simulink model "vehicle_psd"  (R2017a)
settings: Solver=FixedStepDiscrete  StartTime=0.0  StopTime=5e3  FixedStep=abs(Ts)  RelTol=1e-3
InitFcn:
  | if ~exist('Ts')
  |     Ts = 1;
  | end
undefined symbols (not defined in the file or in its folder): elvio_cycle_eu_nedc
libraries: elvio x19
settings Model: Creator=tstef  LastModifiedBy=thomas
settings OptimizationCC: LifeSpan=inf
settings DebuggingCC: SFExecutionAtInitializationDiag=none

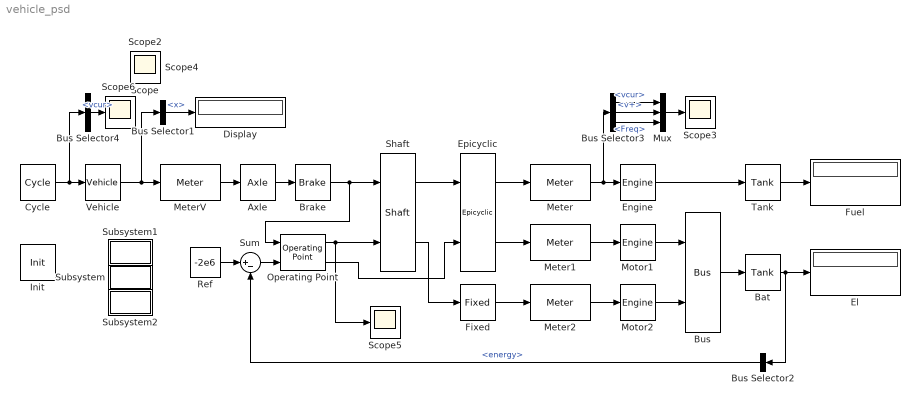
== system vehicle_psd ==
  Axle : elvio/Drive/Axle  radius=0.3  ratio=4  factor=0.1  FromTag1=Axle1  GotoTag1=MeterV1
  Bat : elvio/Drive/Tank  GotoTag1=Bus1
  Brake : elvio/Drive/Brake  Tbrake=5000  FromTag1=Brake1  GotoTag1=Axle1
  Bus : elvio/Drive/Bus  GotoTag1=Motor11  GotoTag2=Motor21  FromTag1=Bus1
  Bus Selector1 : BusSelector  OutputSignals=info.x
  Bus Selector2 : BusSelector  OutputSignals=energy
  Bus Selector3 : BusSelector  OutputSignals=vcur,v+,Freq
  Bus Selector4 : BusSelector  OutputSignals=vcur
  Cycle : elvio/Drive/Cycle  data=elvio_cycle_eu_nedc()
  Display : Display
  El : Display
  Engine : elvio/Drive/Engine  Tmax=110  Tmin=-12  Tfrict=12  Ploss=1000  lossf=1.1  lossnorm=500e3  lossR=0.2  FromTag1=Engine1  GotoTag1=Meter1
  Epicyclic : elvio/Drive/Epicyclic  a=0.4  FromTag1=Epicyclic1  FromTag2=Epicyclic2  GotoTag1=Shaft1
  Fixed : elvio/Drive/Fixed  gear=2  factor=0.1  FromTag1=Fixed1  GotoTag1=Shaft2
  Fuel : Display
  Init : elvio/Drive/Init  Ts0=1
  Meter : elvio/Drive/Meter  FromTag1=Meter1  GotoTag1=Epicyclic1
  Meter1 : elvio/Drive/Meter  FromTag1=Meter11  GotoTag1=Epicyclic2
  Meter2 : elvio/Drive/Meter  FromTag1=Meter21  GotoTag1=Fixed1
  MeterV : elvio/Drive/Meter  FromTag1=MeterV1  GotoTag1=Vehicle1
  Motor1 : elvio/Drive/Engine  Tmax=60  Tmin=-60  Tfrict=0.2  Ploss=100  lossf=0.01  lossnorm=2e6  lossR=0.05  FromTag1=Motor11  GotoTag1=Meter11
  Motor2 : elvio/Drive/Engine  Tmax=60  Tmin=-60  Tfrict=0.2  Ploss=100  lossf=0.01  lossnorm=2e6  lossR=0.05  FromTag1=Motor21  GotoTag1=Meter21
  Mux : Mux  Inputs=3
  Operating Point : elvio/Drive/Operating Point  a=0.4  T=1000  Pk=0.5  Pbias=5e3  Pmin=4e3  vmin=100  vmax=400  Tmin=10  Tmax=80
  Ref : Constant  Value=-2e6
  Scope{,2..6} (6 alike) : Scope
      Scope4 mask Display: disp('1.484e+07')
  Shaft : elvio/Drive/Shaft  FromTag1=Shaft1  FromTag2=Shaft2  GotoTag1=Brake1
  Subsystem : Subsystem
      settings: OpenFcn=elvio_plot_scatter(logsout);
      mask Display: disp('Scatter')
  Subsystem1 : Subsystem
      settings: OpenFcn=elvio_plot_energy(logsout);
      mask Display: disp('Energy')
  Subsystem2 : Subsystem
      settings: OpenFcn=elvio_plot_sources(logsout);
      mask Display: disp('Sources')
  Sum : Sum  Inputs=|+-
  Tank : elvio/Drive/Tank  GotoTag1=Engine1
  Vehicle : elvio/Drive/Vehicle  m=1200  Froll=150  Aeff=0.3:0.025:0.4  n=[1 5]  FromTag1=Vehicle1
  wires:
  Vehicle/1 -> MeterV/1, Bus Selector1/1
  Engine/1 -> Tank/1
  Tank/1 -> Fuel/1
  Operating Point/1 -> Scope5/1, Shaft/2
  Bus/1 -> Bat/1
  Motor1/1 -> Bus/1
  Motor2/1 -> Bus/2
  Shaft/1 -> Epicyclic/1
  Epicyclic/1 -> Meter/1
  Operating Point/2 -> Epicyclic/2
  Bat/1 -> Bus Selector2/1, El/1
  Bus Selector1/1 -> Display/1  "<x>"
  Shaft/2 -> Fixed/1
  Fixed/1 -> Meter2/1
  Epicyclic/2 -> Meter1/1
  Meter1/1 -> Motor1/1
  Meter2/1 -> Motor2/1
  MeterV/1 -> Axle/1
  Bus Selector3/3 -> Mux/3  "<Freq>"
  Bus Selector3/2 -> Mux/2  "<v+>"
  Mux/1 -> Scope3/1
  Meter/1 -> Bus Selector3/1, Engine/1
  Bus Selector3/1 -> Mux/1  "<vcur>"
  Cycle/1 -> Vehicle/1, Bus Selector4/1
  Bus Selector4/1 -> Scope6/1  "<vcur>"
  Axle/1 -> Brake/1
  Brake/1 -> Operating Point/1, Shaft/1
  Ref/1 -> Sum/1
  Bus Selector2/1 -> Sum/2  "<energy>"
  Sum/1 -> Operating Point/2

== system vehicle_psd/Subsystem ==

== system vehicle_psd/Subsystem1 ==

== system vehicle_psd/Subsystem2 ==
